simulink model "model_bez"  (R2017b)
settings: Solver=ode3  StartTime=0.0  StopTime=10.0  FixedStep=0.001  RelTol=1e-3  EnableMultiTasking=on
values from neighbouring files (symbols this model uses):
  K = params(1) * 0.4    [cel.m]
  T = 6    [char_U_V_Az.m]
undefined symbols (not defined in the file or in its folder): offset, psi
settings Model: Creator=Student  LastModifiedBy=Marcin
settings DataIOCC: LimitDataPoints=on  SaveFormat=Array
settings OptimizationCC: LifeSpan=inf
settings DebuggingCC: SFUnexpectedBacktrackingDiag=warning  SFNoUnconditionalDefaultTransitionDiag=warning  SFExecutionAtInitializationDiag=none
settings HardwareCC: ProdBitPerPointer=32  ProdBitPerSizeT=32  ProdBitPerPtrDiffT=32  ProdLargestAtomicFloat=None  ProdIntDivRoundTo=Undefined  ProdEndianess=Unspecified  ProdWordSize=32  ProdHWDeviceType=32-bit Generic
settings ModelReferenceCC: PropagateSignalLabelsOutOfModel=off
settings CodeAppCC: StateflowObjectComments=on
settings GRTTargetCC: TargetLangStandard=C89/C90 (ANSI)  GeneratePreprocessorConditionals=Disable all
settings ConfigComp: CovMetricSettings=dw  CovHtmlReporting=on  CovSaveCumulativeToWorkspaceVar=on  CovSaveSingleToWorkspaceVar=on  CovExternalEMLEnable=off

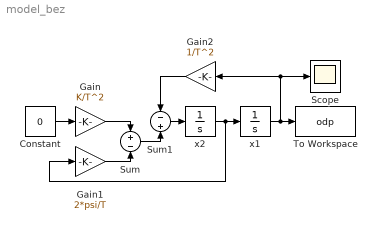
== system model_bez ==
  Constant : Constant  Value=0
  Gain : Gain  Gain=K/T^2
  Gain1 : Gain  Gain=2*psi/T
  Gain2 : Gain  Gain=1/T^2
  Scope : Scope
  Sum : Sum  Inputs=+|-
  Sum1 : Sum  Inputs=-|+
  To Workspace : ToWorkspace  VariableName=odp  SampleTime=-1
  x1 : Integrator  InitialCondition=offset
  x2 : Integrator
  wires:
  Gain/1 -> Sum/1
  Constant/1 -> Gain/1
  x2/1 -> Gain1/1, x1/1
  Sum1/1 -> x2/1
  Gain2/1 -> Sum1/1
  Gain1/1 -> Sum/2
  Sum/1 -> Sum1/2
  x1/1 -> Scope/1, Gain2/1, To Workspace/1
